simulink library "bcm"  (R2021b)
settings: Solver=VariableStepAuto  StartTime=0.0  StopTime=10.0  RelTol=1e-3
undefined symbols (not defined in the file or in its folder): ENUM_ANTITHEFT_ALARM, ENUM_ANTITHEFT_ARM, ENUM_ANTITHEFT_DISARM, ENUM_ANTITHEFT_WAIT, ENUM_GEARPOSNTOCAN_P, ENUM_PDKEYRAWLULOCK_INUNLOCK, ENUM_PDKEYRAWPS_INPS, ENUM_POWERSTA_ON, ENUM_POWERSTA_READY, ENUM_POWERSTA_STANDBY, FALSE, KBCM_ALMBrightnessDark_enum, KBCM_AmbBlue_enum, KBCM_AmbBreathT_ms, KBCM_AmbGreen_enum, KBCM_AmbRed_enum, KBCM_Antitheft_enum_ovrdflg, KBCM_Antitheft_enum_ovrdval, KBCM_APMDoorCtrlSta_flg_ovrdflg, KBCM_APMDoorCtrlSta_flg_ovrdval, KBCM_DelayTSW_flg, KBCM_DiagFLTC_mA, KBCM_DiagFMHT_s, KBCM_DiagFRTC_mA, KBCM_DiagRLTC_mA, KBCM_DiagRRTC_mA, KBCM_DrAPMRetryTimes_cnt, KBCM_DrOpenWdwOT_s, KBCM_DrOpenWdwReady_s, KBCM_ESSOffT_ms, KBCM_ESSOnT_ms, KBCM_IVIRstHoldT_ms, KBCM_IVIRstTriggerT_ms, KBCM_ONDelayT_ms, KBCM_ReDetectT_K, KBCM_RmLampKeep_min, KBCM_RmLpKeyInT_s, KBCM_RmLpKeyMissT_s, KBCM_SlpDebounceTime_s, KBCM_SPTGDetectT_sec, KBCM_SPTGLeave_flg, KBCM_SPTGLeftBound_cm, KBCM_SPTGLeftBoundOut_cm, KBCM_SPTGLowerBound_cm, KBCM_SPTGLowerBoundOut_cm, KBCM_SPTGRightBound_cm, KBCM_SPTGRightBoundOut_cm, KBCM_SPTGTOut_K, KBCM_SPTGUpperBound_cm, KBCM_SPTGUpperBoundOut_cm, KBCM_SPTGWaitDKC_sec, KBCM_TrunSWKeepTime3_s, KBCM_TrunSWKeepTime5_s, KBCM_TrunSWKeepTime7_s, KBCM_USSDis_cm, KBCM_USSFilterT_K, KBCM_WaitAPMPwr_K, KBCM_WdwManualDetT_s, MIN2SEC, TRUE ... (+1)
libraries: simulink x151, hcu_lib x5
(part 1 of 8)
settings Model: Creator=user  LastModifiedBy=FVT22115
settings SolverCC: AlgebraicLoopSolver=TrustRegion
settings DebuggingCC: SFMachineParentedDataDiag=warning

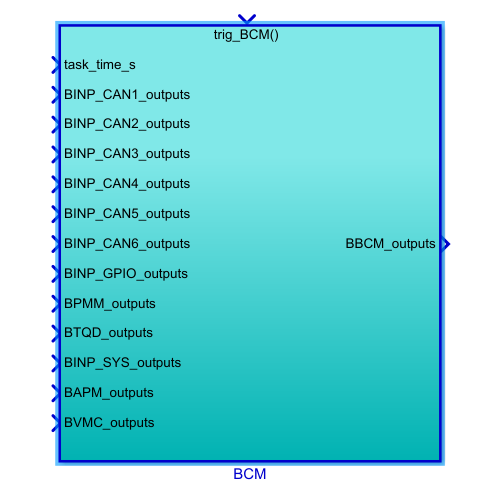
[thumbnail: Simulink's stored preview of the top-level diagram]
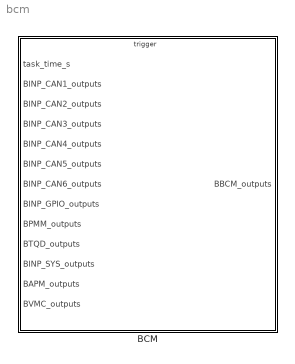
== system bcm ==
  BCM : Subsystem  TreatAsAtomicUnit=on
      settings: RTWSystemCode=Nonreusable function  RTWFcnNameOpts=Use subsystem name  RTWFileNameOpts=Use subsystem name

== system bcm/BCM ==
  task_time_s : Inport
  BINP_CAN1_outputs : Inport  Port=2  OutDataTypeStr=Bus: BINP_CAN1_outputs
  BINP_CAN2_outputs : Inport  Port=3  OutDataTypeStr=Bus: BINP_CAN2_outputs
  BINP_CAN3_outputs : Inport  Port=4  OutDataTypeStr=Bus: BINP_CAN3_outputs
  BINP_CAN4_outputs : Inport  Port=5  OutDataTypeStr=Bus: BINP_CAN4_outputs
  BINP_CAN5_outputs : Inport  Port=6  OutDataTypeStr=Bus: BINP_CAN5_outputs
  BINP_CAN6_outputs : Inport  Port=7  OutDataTypeStr=Bus: BINP_CAN6_outputs
  BINP_GPIO_outputs : Inport  Port=8  OutDataTypeStr=Bus: BINP_GPIO_outputs
  BPMM_outputs : Inport  Port=9  OutDataTypeStr=Bus: BPMM_outputs
  BTQD_outputs : Inport  Port=10  OutDataTypeStr=Bus: BTQD_outputs
  BINP_SYS_outputs : Inport  Port=11  OutDataTypeStr=Bus: BINP_SYS_outputs
  BAPM_outputs : Inport  Port=12  OutDataTypeStr=Bus: BAPM_outputs
  BVMC_outputs : Inport  Port=13  OutDataTypeStr=Bus: BVMC_outputs
  trig_BCM : TriggerPort  TriggerType=function-call  VariantControl=(inherit)
  BCM : Subsystem
  Bus Creator : BusCreator  Inputs=125  OutDataTypeStr=Bus: BBCM_outputs  NonVirtualBus=on
  Bus Selector : BusSelector  OutputSignals=VINP_HoodSW_flg,VINP_TailgateSW_flg,VINP_DrDoorSW_flg,VINP_PsDoorSW_flg,VINP_RLDoorSW_flg,VINP_RRDoorSW_flg,VINP_TrunkHanSW_flg,VINP_HazardSW_flg,VINP_CentralDoorLockSW_flg,VINP_BrakeSWGPIO_flg
  Bus Selector1 : BusSelector  OutputSignals=VPMM_PowerSta_enum
  Bus Selector10 : BusSelector  OutputSignals=VVMC_APSActive_flg
  Bus Selector14 : BusSelector  OutputSignals=VINP_SetUnlockSingle_flg,VINP_IVIStatus_flg,VINP_IVINightModeSta_flg,VINP_HeadLampSW_enum,VINP_RFogLampSW_flg,VINP_FollowMeSW_flg,VINP_IVIRRDefReq_flg,VINP_IVIWIMAINSW_flg,VINP_CANMsgValidIVI2_flg,VINP_CDLUnlockButt_flg,VINP_CDLLockButt_flg,VINP_RoomLampMode_flg,VINP_MFRDNBrightReq_pct,VINP_METERKPHCalcu_kph,VINP_IVIPWModeReq_enum,VINP_AmbLighLowBatAlertSW_flg,VINP_AmbLighSafetyAlertSW_flg,VINP_AmbLightBrightnessSet_enum,VINP_AmbLightDimInDarkSW_flg,VINP_AmbLightSW_flg,VINP_AmbLightWlcmLightSW_flg,VINP_LINKtoDrive_flg,VINP_AmbLightColorSet_enum,VINP_IVIPTGUSStaSW_flg,VINP_LDrvControlCommand_pct,VINP_LPasControlCommand_pct,VINP_LRLDControlCommand_pct,VINP_LRRDControlCommand_pct,VINP_OpenDrOpenWdoSW_flg,VINP_CANMsgValidIVI1_flg,VINP_UserSet_enum,VINP_TurnSwTimeSet_enum,VINP_IVILockSoundSWSta_flg,VINP_AVMParkingmode_enum
  Bus Selector2 : BusSelector  OutputSignals=VINP_PCommandToBCM_enum,VINP_DrLockSta_flg,VINP_CSWDimSw_flg,VINP_CSWPassSWSta_flg,VINP_RLSLampSta_flg,VINP_CSWTurnSwSta_enum,VINP_RLTurnLampC_mA,VINP_RRTurnLampC_mA,VINP_FLTurnLampC_mA,VINP_FRTurnLampC_mA,VINP_MIRRORFOLDSW_flg,VINP_CSWFWasSwSta_enum,VINP_CSWFWipSwSta_enum,VINP_RLSRainSnrWiperCmd_enum,VINP_FWiperAS_flg,VINP_CSWRWipIntSwSta_enum,VINP_RWiperAS_flg,VINP_CSWRWasSWSta_enum,VINP_PTGRDILSta_enum,VINP_RWiperProtection_flg,VINP_FWiperProtection_flg,VINP_PDKeyAreaPTG_enum,VINP_SWCmodeSta_flg,VINP_CANMsgValidDKC1_flg,VINP_CANMsgValidZONEDR1_flg,VINP_CANMsgValidZONEFR1_flg,VINP_PTGInnerSW2_enum,VINP_LDrvValWdwOpened_pct,VINP_LPasValWdwOpened_pct,VINP_LRLDValWdwOpened_pct,VINP_LRRDValWdwOpened_pct,VINP_PDKeyAreaLockUnlock_enum,VINP_PDKeyAreaPS_enum
  Bus Selector3 : BusSelector  OutputSignals=VINP_VehSpeed_kph,VINP_AirBagFailCmd_flg,VINP_ActBrkLampSta_flg,VINP_ESSActive_flg,VINP_SASAngle_Deg
  Bus Selector4 : BusSelector  OutputSignals=VTQD_ShiftGearPosn_enum,VTQD_CrashDetd_flg,VTQD_DiagHCrash_flg,VTQD_ReBrakeLPReq_flg
  Bus Selector5 : BusSelector  OutputSignals=VINP_ReDoorLock_enum,VINP_ReOutsideMirror_enum
  Bus Selector6 : BusSelector  OutputSignals=VINP_FlashAntitheft_enum,VINP_FlashCountAlarm_enum,VINP_FlashMFSWTri_flg,VINP_FlashMirrorFlodPos_flg,VINP_FlashFuelDoorPos_flg,VINP_FlashLockSetting_flg,VINP_FlashMFRDNBrightReq_pct,VINP_FlashRoomLampMode_flg,VINP_FlashWiperFixMode_flg,VINP_FlashIVIPTGUSStaSW_flg,VINP_FlashHoodSW_flg,VINP_FlashTailgateSW_flg,VINP_FlashCTDLockSW_flg,VINP_FlashTailgateHDSW_flg,VINP_FlashAPMDoorControlSta_flg,VINP_FlashfUnlockSingle_flg,VINP_FlashAmbFunEN_enum,VINP_FlashAmbWelEN_enum,VINP_FlashAmbDimEN_enum,VINP_FlashAmbLinkDriSta_enum,VINP_FlashAmbPwrWarnEN_enum,VINP_FlashAmbODAEN_enum,VINP_FlashAmbColorSta1_enum,VINP_FlashAmbColorSta2_enum,VINP_FlashAmbColorSta3_enum,VINP_FlashAmbColorSta4_enum,VINP_FlashAmbColorSta5_enum,VINP_FlashAmbColorSta7_enum,VINP_FlashAmbBrightnessSta1_enum,VINP_FlashAmbBrightnessSta2_enum,VINP_FlashAmbBrightnessSta3_enum,VINP_FlashAmbBrightnessSta4_enum,VINP_FlashAmbBrightnessSta5_enum,VINP_FlashAmbBrightnessSta7_enum
  Bus Selector7 : BusSelector  OutputSignals=VAPM_PASDRMR_cm,VAPM_PASDRML_cm
  Bus Selector8 : BusSelector  OutputSignals=VINP_SRRODAWarnR_enum,VINP_SRRODAWarnL_enum,VINP_SRRBSDWarnR_enum,VINP_SRRBSDWarnL_enum,VINP_LeftTurnLightReq_flg,VINP_RightTurnLightReq_flg,VINP_ForceLowBeam_enum,VINP_HazardWarningReq_flg
  Bus Selector9 : BusSelector  OutputSignals=VINP_HVBattSOCDis_pct,VINP_CSW2DimSwSta_flg,VINP_CSW2PassSWSta_flg,VINP_CSW2FWipSwSta_enum,VINP_CSW2FWasSwSta_enum,VINP_CSW2TurnSwSta_enum,VINP_CSW2RWipWasSwSta_enum
  Ground{1..2,6..12,14} (10 alike) : Ground
  Model Info : simulink/Model-Wide Utilities/Model Info  Frame=on  DisplayStringWithTags=$Id: pmm.mdl 130 2021-02-08 12:40:01Z Shawn $  HorizontalTextAlignment=Center  LeftAlignmentValue=0.5
  BBCM_outputs : Outport  OutDataTypeStr=Bus: BBCM_outputs  VectorParamsAs1DForOutWhenUnconnected=off
  wires:
  BPMM_outputs/1 -> Bus Selector1/1
  BINP_CAN4_outputs/1 -> [BINP_CAN4_outputs]
  BINP_CAN1_outputs/1 -> [BINP_CAN1_outputs]
  [BINP_CAN1_outputs] -> Bus Selector3/1
  BINP_GPIO_outputs/1 -> [BINP_GPIO_outputs]
  [BINP_GPIO_outputs] -> Bus Selector/1
  BINP_CAN2_outputs/1 -> [BINP_CAN2_outputs]
  BINP_CAN5_outputs/1 -> [BINP_CAN5_outputs]
  [BINP_CAN2_outputs] -> Bus Selector14/1
  BTQD_outputs/1 -> Bus Selector4/1
  Bus Selector3/2 -> BCM/3(VINP_AirBagFailCmd_flg)  "<VINP_AirBagFailCmd_flg>"
  Bus Selector3/1 -> BCM/2(VINP_VehSpeed_kph)  "<VINP_VehSpeed_kph>"
  [BINP_CAN4_outputs] -> Bus Selector2/1
  [BINP_CAN5_outputs] -> Bus Selector5/1
  Bus Selector14/9 -> BCM/23(VINP_CANMsgValidIVI2_flg)  "<VINP_CANMsgValidIVI2_flg>"
  Bus Selector14/2 -> BCM/16(VINP_IVIStatus_flg)  "<VINP_IVIStatus_flg>"
  Bus Selector14/3 -> BCM/17(VINP_IVINightModeSta_flg)  "<VINP_IVINightModeSta_flg>"
  Bus Selector14/4 -> BCM/18(VINP_HeadLampSW_enum)  "<VINP_HeadLampSW_enum>"
  Bus Selector14/5 -> BCM/19(VINP_RFogLampSW_flg)  "<VINP_RFogLampSW_flg>"
  Bus Selector14/6 -> BCM/20(VINP_FollowMeSW_flg)  "<VINP_FollowMeSW_flg>"
  Bus Selector14/1 -> BCM/15(VINP_SetUnlockSingle_flg)  "<VINP_SetUnlockSingle_flg>"
  Bus Selector14/7 -> BCM/21(VINP_IVIRRDefReq_flg)  "<VINP_IVIRRDefReq_flg>"
  Bus Selector14/8 -> BCM/22(VINP_IVIWIMAINSW_flg)  "<VINP_IVIWIMAINSW_flg>"
  Bus Selector14/10 -> BCM/24(VINP_CDLUnlockButt_flg)  "<VINP_CDLUnlockButt_flg>"
  Bus Selector14/11 -> BCM/25(VINP_CDLLockButt_flg)  "<VINP_CDLLockButt_flg>"
  Bus Selector14/12 -> BCM/26(VINP_RoomLampMode_flg)  "<VINP_RoomLampMode_flg>"
  Bus Selector14/13 -> BCM/27(VINP_MFRDNBrightReq_pct)  "<VINP_MFRDNBrightReq_pct>"
  Bus Selector14/14 -> BCM/28(VINP_METERKPHCalcu_kph)  "<VINP_METERKPHCalcu_kph>"
  Bus Selector14/15 -> BCM/29(VINP_IVIPWModeReq_enum)  "<VINP_IVIPWModeReq_enum>"
  task_time_s/1 -> BCM/1(task_time_s)
  BINP_SYS_outputs/1 -> Bus Selector6/1  "BINP_SYS_output"
  BAPM_outputs/1 -> Bus Selector7/1  "BAPM_outputs"
  BINP_CAN6_outputs/1 -> [BINP_CAN6_outputs]
  [BINP_CAN6_outputs] -> Bus Selector8/1
  Bus Selector8/5 -> BCM/11(VINP_LeftTurnReq_flg)  "<VINP_LeftTurnLightReq_flg>"
  Bus Selector8/6 -> BCM/12(VINP_RightTurnReq_flg)  "<VINP_RightTurnLightReq_flg>"
  Bus Selector8/7 -> BCM/13(VINP_ForceLowBeam_enum)  "<VINP_ForceLowBeam_enum>"
  Bus Selector8/8 -> BCM/14(VINP_HazardWarningReq_flg)  "<VINP_HazardWarningReq_flg>"
  Bus Selector3/3 -> BCM/4(VINP_ActBrkLampSta_flg)  "<VINP_ActBrkLampSta_flg>"
  Bus Selector3/4 -> BCM/5(VINP_ESSActive_flg)  "<VINP_ESSActive_flg>"
  Bus Selector8/1 -> BCM/7(VINP_SRRODAWarnR_enum)  "<VINP_SRRODAWarnR_enum>"
  Bus Selector8/2 -> BCM/8(VINP_SRRODAWarnL_enum)  "<VINP_SRRODAWarnL_enum>"
  Bus Selector8/3 -> BCM/9(VINP_SRRBSDWarnR_enum)  "<VINP_SRRBSDWarnR_enum>"
  Bus Selector8/4 -> BCM/10(VINP_SRRBSDWarnL_enum)  "<VINP_SRRBSDWarnL_enum>"
  Bus Selector14/24 -> BCM/38(VINP_IVIPTGUSStaSW_flg)  "<VINP_IVIPTGUSStaSW_flg>"
  Bus Selector14/25 -> BCM/39(VINP_LDrvControlCommand_pct)  "<VINP_LDrvControlCommand_pct>"
  Bus Selector14/26 -> BCM/40(VINP_LPasControlCommand_pct)  "<VINP_LPasControlCommand_pct>"
  Bus Selector14/27 -> BCM/41(VINP_LRLDControlCommand_pct)  "<VINP_LRLDControlCommand_pct>"
  Bus Selector14/28 -> BCM/42(VINP_LRRDControlCommand_pct)  "<VINP_LRRDControlCommand_pct>"
  Bus Selector14/29 -> BCM/43(VINP_OpenDrOpenWdoSW_flg)  "<VINP_OpenDrOpenWdoSW_flg>"
  Bus Selector2/1 -> BCM/56(VINP_PCommandToBCM_enum)  "<VINP_PCommandToBCM_enum>"
  Bus Selector2/2 -> BCM/57(VINP_DrLockSta_flg)  "<VINP_DrLockSta_flg>"
  Bus Selector2/3 -> BCM/58(VINP_CSWDimSw_flg)  "<VINP_CSWDimSw_flg>"
  Bus Selector2/4 -> BCM/59(VINP_CSWPassSWSta_flg)  "<VINP_CSWPassSWSta_flg>"
  Bus Selector2/5 -> BCM/60(VINP_RLSLampSta_flg)  "<VINP_RLSLampSta_flg>"
  Bus Selector2/6 -> BCM/61(VINP_CSWTurnSWSta_enum)  "<VINP_CSWTurnSwSta_enum>"
  Bus Selector2/7 -> BCM/62(VINP_RLTurnLampC_mA)  "<VINP_RLTurnLampC_mA>"
  Bus Selector2/8 -> BCM/63(VINP_RRTurnLampC_mA)  "<VINP_RRTurnLampC_mA>"
  Bus Selector2/9 -> BCM/64(VINP_FLTurnLampC_mA)  "<VINP_FLTurnLampC_mA>"
  Bus Selector2/10 -> BCM/65(VINP_FRTurnLampC_mA)  "<VINP_FRTurnLampC_mA>"
  Bus Selector2/11 -> BCM/66(VINP_MIRRORFOLDSW_flg)  "<VINP_MIRRORFOLDSW_flg>"
  Bus Selector2/12 -> BCM/67(VINP_CSWFWasSWSta_enum)  "<VINP_CSWFWasSwSta_enum>"
  Bus Selector2/13 -> BCM/68(VINP_CSWFWipSWSta_enum)  "<VINP_CSWFWipSwSta_enum>"
  Bus Selector2/14 -> BCM/69(VINP_RLSRainSnrWiperCmd_enum)  "<VINP_RLSRainSnrWiperCmd_enum>"
  Bus Selector2/15 -> BCM/70(VINP_FWiperAS_flg)  "<VINP_FWiperAS_flg>"
  Bus Selector2/16 -> BCM/71(VINP_CSWRWipIntSwSta_enum)  "<VINP_CSWRWipIntSwSta_enum>"
  Bus Selector2/17 -> BCM/72(VINP_RWiperAS_flg)  "<VINP_RWiperAS_flg>"
  Bus Selector2/18 -> BCM/73(VINP_CSWRWasSWSta_enum)  "<VINP_CSWRWasSWSta_enum>"
  Bus Selector2/19 -> BCM/74(VINP_PTGRDILsta_enum)  "<VINP_PTGRDILSta_enum>"
  Bus Selector2/20 -> BCM/75(VINP_RWiperProtection_flg)  "<VINP_RWiperProtection_flg>"
  Bus Selector2/21 -> BCM/76(VINP_FWiperProtection_flg)  "<VINP_FWiperProtection_flg>"
  Bus Selector2/22 -> BCM/77(VINP_PDKeyAreaPTG_enum)  "<VINP_PDKeyAreaPTG_enum>"
  Bus Selector2/23 -> BCM/78(VINP_SWCmodeSta_flg)  "<VINP_SWCmodeSta_flg>"
  Bus Selector2/24 -> BCM/79(VINP_CANMsgValidDKC1_flg)  "<VINP_CANMsgValidDKC1_flg>"
  Bus Selector2/25 -> BCM/80(VINP_CANMsgValidGWZoneDR1_flg)  "<VINP_CANMsgValidZONEDR1_flg>"
  Bus Selector2/26 -> BCM/81(VINP_CANMsgValidGWZoneFR1_flg)  "<VINP_CANMsgValidZONEFR1_flg>"
  Bus Selector2/27 -> BCM/82(VINP_PTGInnerSW2_enum)  "<VINP_PTGInnerSW2_enum>"
  Bus Selector2/28 -> BCM/83(VINP_LDrvValWdwOpened_pct)  "<VINP_LDrvValWdwOpened_pct>"
  Bus Selector2/29 -> BCM/84(VINP_LPasValWdwOpened_pct)  "<VINP_LPasValWdwOpened_pct>"
  Bus Selector2/30 -> BCM/85(VINP_LRLDValWdwOpened_pct)  "<VINP_LRLDValWdwOpened_pct>"
  Bus Selector2/31 -> BCM/86(VINP_LRRDValWdwOpened_pct)  "<VINP_LRRDValWdwOpened_pct>"
  Bus Selector2/32 -> BCM/87(VINP_PDKeyAreaLockUnlock_enum)  "<VINP_PDKeyAreaLockUnlock_enum>"
  Bus Selector2/33 -> BCM/88(VINP_PDKeyAreaPS_enum)  "<VINP_PDKeyAreaPS_enum>"
  Bus Selector5/1 -> BCM/89(VINP_ReDoorLock_enum)  "<VINP_ReDoorLock_enum>"
  Bus Selector5/2 -> BCM/90(VINP_ReOutsideMirror_enum)  "<VINP_ReOutsideMirror_enum>"
  Bus Selector/1 -> BCM/91(VINP_HoodSW_flg)  "<VINP_HoodSW_flg>"
  Bus Selector/2 -> BCM/92(VINP_TailgateSW_flg)  "<VINP_TailgateSW_flg>"
  Bus Selector/3 -> BCM/93(VINP_DrDoorSW_flg)  "<VINP_DrDoorSW_flg>"
  Bus Selector/4 -> BCM/94(VINP_PsDoorSW_flg)  "<VINP_PsDoorSW_flg>"
  Bus Selector/5 -> BCM/95(VINP_RLDoorSW_flg)  "<VINP_RLDoorSW_flg>"
  Bus Selector/6 -> BCM/96(VINP_RRDoorSW_flg)  "<VINP_RRDoorSW_flg>"
  Bus Selector/7 -> BCM/97(VINP_TrunkHanSW_flg)  "<VINP_TrunkHanSW_flg>"
  Bus Selector/8 -> BCM/98(VINP_HazardSW_flg)  "<VINP_HazardSW_flg>"
  Bus Selector/9 -> BCM/99(VINP_CentralDoorLockSW_flg)  "<VINP_CentralDoorLockSW_flg>"
  Bus Selector/10 -> BCM/100(VINP_BrakeSWGPIO_flg)  "<VINP_BrakeSWGPIO_flg>"
  Bus Selector1/1 -> BCM/101(VPMM_PwrSta_enum)  "<VPMM_PowerSta_enum>"
  Bus Selector4/1 -> BCM/102(VTQD_ShiftGearPosn_enum)  "<VTQD_ShiftGearPosn_enum>"
  Bus Selector4/2 -> BCM/103(VTQD_CrashDetd_flg)  "<VTQD_CrashDetd_flg>"
  Bus Selector4/3 -> BCM/104(VTQD_DiagHCrash_flg)  "<VTQD_DiagHCrash_flg>"
  Bus Selector4/4 -> BCM/105(VTQD_ReBrakeLPReq_flg)  "<VTQD_ReBrakeLPReq_flg>"
  Bus Selector6/1 -> BCM/106(VINP_FlashAntitheft_enum)  "<VINP_FlashAntitheft_enum>"
  Bus Selector6/2 -> BCM/107(VINP_FlashCountAlarm_enum)  "<VINP_FlashCountAlarm_enum>"
  Bus Selector6/3 -> BCM/108(VINP_FlashMFSWTri_flg)  "<VINP_FlashMFSWTri_flg>"
  Bus Selector6/4 -> BCM/109(VINP_FlashMirrorFlodPos)  "<VINP_FlashMirrorFlodPos_flg>"
  Bus Selector6/5 -> BCM/110(VINP_FlashFuelDoorPos)  "<VINP_FlashFuelDoorPos_flg>"
  Bus Selector6/6 -> BCM/111(VINP_FlashLockSetting_flg)  "<VINP_FlashLockSetting_flg>"
  Bus Selector6/7 -> BCM/112(VINP_FlashMFRDNBrightReq_pct)  "<VINP_FlashMFRDNBrightReq_pct>"
  Bus Selector6/8 -> BCM/113(VINP_FlashRoomLampMode_flg)  "<VINP_FlashRoomLampMode_flg>"
  Bus Selector6/9 -> BCM/114(VINP_FlashWiperFixMode_flg)  "<VINP_FlashWiperFixMode_flg>"
  Bus Selector6/10 -> BCM/115(VINP_FlashIVIPTGUSStaSW_flg)  "<VINP_FlashIVIPTGUSStaSW_flg>"
  Bus Selector6/11 -> BCM/116(VINP_FlashHoodSW_flg)  "<VINP_FlashHoodSW_flg>"
  Bus Selector6/12 -> BCM/117(VINP_FlashTailgateSW_flg)  "<VINP_FlashTailgateSW_flg>"
  Bus Selector6/13 -> BCM/118(VINP_FlashCTDLockSW_flg)  "<VINP_FlashCTDLockSW_flg>"
  Bus Selector6/14 -> BCM/119(VINP_FlashTailgateHDSW_flg)  "<VINP_FlashTailgateHDSW_flg>"
  Bus Selector6/15 -> BCM/120(VINP_FlashAPMDoorControlSta_flg)  "<VINP_FlashAPMDoorControlSta_flg>"
  Ground1/1 -> BCM/142(VINP_DiagFMHT_s)
  Ground9/1 -> BCM/143(VINP_DiagFLTC_mA)
  Ground7/1 -> BCM/144(VINP_DiagFRTC_mA)
  Ground10/1 -> BCM/146(VINP_DiagRRTC_mA)
  Ground8/1 -> BCM/145(VINP_DiagRLTC_mA)
  Ground2/1 -> BCM/141(VINP_DiagDRLOFF_flg)
  Ground6/1 -> BCM/140(VINP_funAuto_flg)
  Bus Selector7/1 -> BCM/147(VAPM_PASDRMR_cm)  "<VAPM_PASDRMR_cm>"
  Bus Selector7/2 -> BCM/148(VAPM_PASDRML_cm)  "<VAPM_PASDRML_cm>"
  Ground11/1 -> BCM/151(VDDM_HVRlyOpCFS_flg)
  Ground12/1 -> BCM/152(VDDM_MCUActCFS_flg)
  Ground14/1 -> BCM/150(VINP_RRDefSta_flg)
  Bus Creator/1 -> BBCM_outputs/1
  BCM/1(VBCM_AntitheftSta_enum) -> Bus Creator/1
  BCM/2(VBCM_TailgateRemote_enum) -> Bus Creator/2
  BCM/3(VBCM_HornCtrl_flg) -> Bus Creator/3
  BCM/4(VBCM_AllDoorSW_flg) -> Bus Creator/4
  BCM/5(VBCM_BCMDoorLockSta_flg) -> Bus Creator/5
  BCM/6(VBCM_AntitheftSeatFlod_flg) -> Bus Creator/6
  BCM/7(VBCM_HoodSW_flg) -> Bus Creator/7
  BCM/8(VBCM_TailgateSW_flg) -> Bus Creator/8
  BCM/9(VBCM_DrDoorSW_flg) -> Bus Creator/9
  BCM/10(VBCM_PsDoorSW_flg) -> Bus Creator/10
  BCM/11(VBCM_RLDoorSW_flg) -> Bus Creator/11
  BCM/12(VBCM_RRDoorSW_flg) -> Bus Creator/12
  BCM/13(VBCM_LockSetting_flg) -> Bus Creator/13
  BCM/14(VBCM_FrChargingDoorCtrl_enum) -> Bus Creator/14
  BCM/15(VBCM_RrChargingDoorCtrl_enum) -> Bus Creator/15
  BCM/16(VBCM_CrashSDetd_flg) -> Bus Creator/16
  BCM/17(VBCM_CTDCtrl_enum) -> Bus Creator/17
  BCM/18(VBCM_DoorLockIND_flg) -> Bus Creator/18
  BCM/19(VBCM_CTDLockSW_flg) -> Bus Creator/19
  BCM/20(VBCM_Dimmer_pct) -> Bus Creator/20
  BCM/21(VBCM_DimmerEN_flg) -> Bus Creator/21
  BCM/22(VBCM_PosLamp_flg) -> Bus Creator/22
  BCM/23(VBCM_LBeam_flg) -> Bus Creator/23
  BCM/24(VBCM_HBeam_flg) -> Bus Creator/24
  BCM/25(VBCM_RrFogLamp_flg) -> Bus Creator/25
  BCM/26(VBCM_BrakeLamp_flg) -> Bus Creator/26
  BCM/27(VBCM_ReverseLamp_flg) -> Bus Creator/27
  BCM/28(VBCM_LDRL_flg) -> Bus Creator/28
  BCM/29(VBCM_RDRL_flg) -> Bus Creator/29
  BCM/30(VBCM_LBSD_flg) -> Bus Creator/30
  BCM/31(VBCM_RBSD_flg) -> Bus Creator/31
  BCM/32(VBCM_HazardSW_flg) -> Bus Creator/32
  BCM/33(VBCM_LTurnLP_flg) -> Bus Creator/33
  BCM/34(VBCM_RTurnLP_flg) -> Bus Creator/34
  BCM/35(VBCM_BCMBuzzerReq_flg) -> Bus Creator/35
  BCM/36(VBCM_MirrorCtrl_enum) -> Bus Creator/36
  BCM/37(VBCM_MirrorDefog_flg) -> Bus Creator/37
  BCM/38(VBCM_RrDefog_flg) -> Bus Creator/38
  BCM/39(VBCM_RoomLampH_flg) -> Bus Creator/39
  BCM/40(VBCM_RoomLampL_flg) -> Bus Creator/40
  BCM/41(VBCM_TrunkRel_flg) -> Bus Creator/41
  BCM/42(VBCM_TailgateHDSW_flg) -> Bus Creator/42
  BCM/43(VBCM_FWiperL_flg) -> Bus Creator/43
  BCM/44(VBCM_FWiperH_flg) -> Bus Creator/44
  BCM/45(VBCM_RWiper_flg) -> Bus Creator/45
  BCM/46(VBCM_WasherCtrl_enum) -> Bus Creator/46
  BCM/47(VBCM_WiperFixMode_flg) -> Bus Creator/47
  BCM/48(VBCM_SleepReq_flg) -> Bus Creator/48
  BCM/49(VBCM_AmbLightBreath1_enum) -> Bus Creator/49
  BCM/50(VBCM_AmbLightBreath2_enum) -> Bus Creator/50
  BCM/51(VBCM_AmbLightBreath3_enum) -> Bus Creator/51
  BCM/52(VBCM_AmbLightBreath4_enum) -> Bus Creator/52
  BCM/53(VBCM_AmbLightBreath5_enum) -> Bus Creator/53
  BCM/54(VBCM_AmbLightBreath6_enum) -> Bus Creator/54
  BCM/55(VBCM_AmbLightBrightness1_enum) -> Bus Creator/55
  BCM/56(VBCM_AmbLightBrightness2_enum) -> Bus Creator/56
  BCM/57(VBCM_AmbLightBrightness3_enum) -> Bus Creator/57
  BCM/58(VBCM_AmbLightBrightness4_enum) -> Bus Creator/58
  BCM/59(VBCM_AmbLightBrightness5_enum) -> Bus Creator/59
  BCM/60(VBCM_AmbLightBrightness6_enum) -> Bus Creator/60
  BCM/61(VBCM_AmbLightColor1_enum) -> Bus Creator/61
  BCM/62(VBCM_AmbLightColor2_enum) -> Bus Creator/62
  BCM/63(VBCM_AmbLightColor3_enum) -> Bus Creator/63
  BCM/64(VBCM_AmbLightColor4_enum) -> Bus Creator/64
  BCM/65(VBCM_AmbLightColor5_enum) -> Bus Creator/65
  BCM/66(VBCM_AmbLightColor6_enum) -> Bus Creator/66
  BCM/67(VBCM_LampPwr_flg) -> Bus Creator/67
  BCM/68(VBCM_SPTGDet_flg) -> Bus Creator/68
  BCM/69(VBCM_APSOpenPTG_flg) -> Bus Creator/69
  BCM/70(VBCM_FollowMe_flg) -> Bus Creator/70
  BCM/71(VBCM_IVIRST_flg) -> Bus Creator/71
  BCM/72(VBCM_CountAlarm_enum) -> Bus Creator/72
  BCM/73(VBCM_MFSWTri_flg) -> Bus Creator/73
  BCM/74(VBCM_MirrorFlodPos_flg) -> Bus Creator/74
  BCM/75(VBCM_FuelDoorPos_flg) -> Bus Creator/75
  BCM/76(VBCM_MFRDNBrightReq_pct) -> Bus Creator/76
  BCM/77(VBCM_RoomLampMode_flg) -> Bus Creator/77
  BCM/78(VBCM_IVIPTGUSStaSW_flg) -> Bus Creator/78
  BCM/79(VBCM_PTGInnerSW2_enum) -> Bus Creator/79
  BCM/80(VBCM_DiagHCrash_flg) -> Bus Creator/80
  BCM/81(VBCM_DiagFLTS_flg) -> Bus Creator/81
  BCM/82(VBCM_DiagFRTS_flg) -> Bus Creator/82
  BCM/83(VBCM_DiagRLTS_flg) -> Bus Creator/83
  BCM/84(VBCM_DiagRRTS_flg) -> Bus Creator/84
  BCM/85(VBCM_LDrvCtrlCmd_pct) -> Bus Creator/85
  BCM/86(VBCM_LPasCtrlCmd_pct) -> Bus Creator/86
  BCM/87(VBCM_LRLDCtrlCmd_pct) -> Bus Creator/87
  BCM/88(VBCM_LRRDCtrlCmd_pct) -> Bus Creator/88
  BCM/89(VBCM_APMDoorControlSta_flg) -> Bus Creator/89
  Bus Selector14/22 -> BCM/36(VINP_LINKtoDRIVE_flg)  "<VINP_LINKtoDrive_flg>"
  Bus Selector14/23 -> BCM/37(VINP_AmbLightColorSet_enum)  "<VINP_AmbLightColorSet_enum>"
  Bus Selector14/21 -> BCM/35(VINP_AmbLightWlcmLightSW_flg)  "<VINP_AmbLightWlcmLightSW_flg>"
  Bus Selector14/20 -> BCM/34(VINP_AmbLightSW_flg)  "<VINP_AmbLightSW_flg>"
  Bus Selector14/19 -> BCM/33(VINP_AmbLightDimInDarkSW_flg)  "<VINP_AmbLightDimInDarkSW_flg>"
  Bus Selector14/18 -> BCM/32(VINP_AmbLightBrightnessSet_enum)  "<VINP_AmbLightBrightnessSet_enum>"
  Bus Selector14/17 -> BCM/31(VINP_AmbLighSafetyAlertSW_flg)  "<VINP_AmbLighSafetyAlertSW_flg>"
  Bus Selector14/16 -> BCM/30(VINP_AmbLighLowBatAlertSW_flg)  "<VINP_AmbLighLowBatAlertSW_flg>"
  BINP_CAN3_outputs/1 -> [BINP_CAN3_outputs]
  [BINP_CAN3_outputs] -> Bus Selector9/1
  Bus Selector9/1 -> BCM/49(VINP_HVBattSOCDis_pct)  "<VINP_HVBattSOCDis_pct>"
  BCM/90(VBCM_AmbFunEN_flg) -> Bus Creator/90
  BCM/91(VBCM_AmbWelEN_flg) -> Bus Creator/91
  BCM/92(VBCM_AmbDimEN_flg) -> Bus Creator/92
  BCM/93(VBCM_AmbLinkDriSta_flg) -> Bus Creator/93
  BCM/94(VBCM_AmbPwrWarnEN_flg) -> Bus Creator/94
  BCM/95(VBCM_AmbODAEN_flg) -> Bus Creator/95
  BCM/96(VBCM_AmbColorSta_enum) -> Bus Creator/96
  BCM/97(VBCM_AmbBrightSta_enum) -> Bus Creator/97
  BCM/98(VBCM_LockAlarm_enum) -> Bus Creator/98
  Bus Selector14/30 -> BCM/44(VINP_CANMsgValidIVI1_flg)  "<VINP_CANMsgValidIVI1_flg>"
  BCM/99(VBCM_ATCtrl_enum) -> Bus Creator/99
  BCM/100(VBCM_fUnlockSingle_flg) -> Bus Creator/100
  BCM/101(VBCM_UserNow_enum) -> Bus Creator/101
  BCM/102(VBCM_AmbFunENFlash_enum) -> Bus Creator/102
  BCM/103(VBCM_AmbWelENFlash_enum) -> Bus Creator/103
  BCM/104(VBCM_AmbDimENFlash_enum) -> Bus Creator/104
  BCM/105(VBCM_AmbLinkDriStaFlash_enum) -> Bus Creator/105
  BCM/106(VBCM_AmbPwrWarnENFlash_enum) -> Bus Creator/106
  BCM/107(VBCM_AmbODAENFlash_enum) -> Bus Creator/107
  BCM/108(VBCM_AmbColorSta1_enum) -> Bus Creator/108
  BCM/109(VBCM_AmbColorSta2_enum) -> Bus Creator/109
  BCM/110(VBCM_AmbColorSta3_enum) -> Bus Creator/110
  BCM/111(VBCM_AmbColorSta4_enum) -> Bus Creator/111
  BCM/112(VBCM_AmbColorSta5_enum) -> Bus Creator/112
  BCM/113(VBCM_AmbColorSta7_enum) -> Bus Creator/113
  BCM/114(VBCM_AmbBrightnessSta1_enum) -> Bus Creator/114
  BCM/115(VBCM_AmbBrightnessSta2_enum) -> Bus Creator/115
  BCM/116(VBCM_AmbBrightnessSta3_enum) -> Bus Creator/116
  BCM/117(VBCM_AmbBrightnessSta4_enum) -> Bus Creator/117
  BCM/118(VBCM_AmbBrightnessSta5_enum) -> Bus Creator/118
  BCM/119(VBCM_AmbBrightnessSta7_enum) -> Bus Creator/119
  Bus Selector6/16 -> BCM/121(VINP_FlashfUnlockSingle_flg)  "<VINP_FlashfUnlockSingle_flg>"
  Bus Selector6/17 -> BCM/122(VINP_FlashAmbFunEN_enum)  "<VINP_FlashAmbFunEN_enum>"
  Bus Selector6/18 -> BCM/123(VINP_FlashAmbWelEN_enum)  "<VINP_FlashAmbWelEN_enum>"
  Bus Selector6/19 -> BCM/124(VINP_FlashAmbDimEN_enum)  "<VINP_FlashAmbDimEN_enum>"
  Bus Selector6/20 -> BCM/125(VINP_FlashAmbLinkDriSta_enum)  "<VINP_FlashAmbLinkDriSta_enum>"
  Bus Selector6/21 -> BCM/126(VINP_FlashAmbPwrWarnEN_enum)  "<VINP_FlashAmbPwrWarnEN_enum>"
  Bus Selector6/22 -> BCM/127(VINP_FlashAmbODAEN_enum)  "<VINP_FlashAmbODAEN_enum>"
  Bus Selector6/23 -> BCM/128(VINP_FlashAmbColorSta1_enum)  "<VINP_FlashAmbColorSta1_enum>"
  Bus Selector6/24 -> BCM/129(VINP_FlashAmbColorSta2_enum)  "<VINP_FlashAmbColorSta2_enum>"
  Bus Selector6/25 -> BCM/130(VINP_FlashAmbColorSta3_enum)  "<VINP_FlashAmbColorSta3_enum>"
  Bus Selector6/26 -> BCM/131(VINP_FlashAmbColorSta4_enum)  "<VINP_FlashAmbColorSta4_enum>"
  Bus Selector6/27 -> BCM/132(VINP_FlashAmbColorSta5_enum)  "<VINP_FlashAmbColorSta5_enum>"
  Bus Selector6/28 -> BCM/133(VINP_FlashAmbColorSta7_enum)  "<VINP_FlashAmbColorSta7_enum>"
  Bus Selector6/29 -> BCM/134(VINP_FlashAmbBrightnessSta1_enum)  "<VINP_FlashAmbBrightnessSta1_enum>"
  Bus Selector6/30 -> BCM/135(VINP_FlashAmbBrightnessSta2_enum)  "<VINP_FlashAmbBrightnessSta2_enum>"
  Bus Selector6/31 -> BCM/136(VINP_FlashAmbBrightnessSta3_enum)  "<VINP_FlashAmbBrightnessSta3_enum>"
  Bus Selector6/32 -> BCM/137(VINP_FlashAmbBrightnessSta4_enum)  "<VINP_FlashAmbBrightnessSta4_enum>"
  Bus Selector6/33 -> BCM/138(VINP_FlashAmbBrightnessSta5_enum)  "<VINP_FlashAmbBrightnessSta5_enum>"
  Bus Selector6/34 -> BCM/139(VINP_FlashAmbBrightnessSta7_enum)  "<VINP_FlashAmbBrightnessSta7_enum>"
  Bus Selector14/31 -> BCM/45(VINP_UserSet_enum)  "<VINP_UserSet_enum>"
  BCM/120(VBCM_HazardIND_flg) -> Bus Creator/120
  BCM/121(VBCM_DimSwSta_flg) -> Bus Creator/121
  BCM/122(VBCM_PassSWSta_flg) -> Bus Creator/122
  BCM/123(VBCM_FWipSwSta_enum) -> Bus Creator/123
  BCM/124(VBCM_FWasSwSta_enum) -> Bus Creator/124
  BCM/125(VBCM_TurnSwSta_enum) -> Bus Creator/125
  Bus Selector3/5 -> BCM/6(VINP_SASAngle_Deg)  "<VINP_SASAngle_Deg>"
  Bus Selector14/32 -> BCM/46(VINP_TurnSwTimeSet_enum)  "<VINP_TurnSwTimeSet_enum>"
  Bus Selector9/2 -> BCM/50(VINP_CSW2DimSwSta_flg)  "<VINP_CSW2DimSwSta_flg>"
  Bus Selector9/3 -> BCM/51(VINP_CSW2PassSWSta_flg)  "<VINP_CSW2PassSWSta_flg>"
  Bus Selector9/4 -> BCM/52(VINP_CSW2FWipSwSta_enum)  "<VINP_CSW2FWipSwSta_enum>"
  Bus Selector9/5 -> BCM/53(VINP_CSW2FWasSwSta_enum)  "<VINP_CSW2FWasSwSta_enum>"
  Bus Selector9/6 -> BCM/54(VUNP_CSW2TurnSwSta_enum)  "<VINP_CSW2TurnSwSta_enum>"
  Bus Selector9/7 -> BCM/55(VINP_CSW2RWipWasSwSta_enum)  "<VINP_CSW2RWipWasSwSta_enum>"
  Bus Selector14/33 -> BCM/47(VINP_IVILockSoundSWSta_flg)  "<VINP_IVILockSoundSWSta_flg>"
  Bus Selector14/34 -> BCM/48(VINP_AVMparkingmode_enum)  "<VINP_AVMParkingmode_enum>"
  BVMC_outputs/1 -> Bus Selector10/1  "BVMC_outputs"
  Bus Selector10/1 -> BCM/149(VINP_APSActive_flg)  "<VVMC_APSActive_flg>"
